simulink model "untitled"  (R2020a)
settings: Solver=VariableStepAuto  StartTime=0.0  StopTime=10.0  RelTol=1e-3
libraries: simulink_extras x1
settings Model: Creator=jiho  LastModifiedBy=jiho

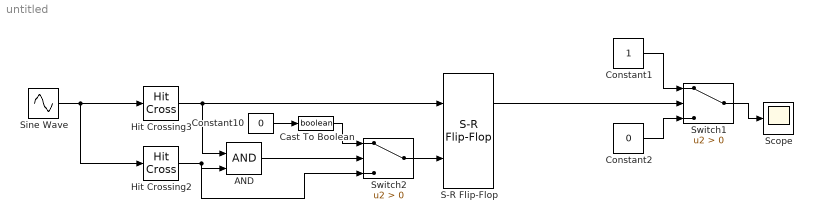
== system untitled ==
  AND : Logic  IconShape=distinctive  AllPortsSameDT=off  OutDataTypeStr=boolean
  Cast To Boolean : DataTypeConversion  OutDataTypeStr=boolean
  Constant1 : Constant
  Constant10 : Constant  Value=0
  Constant2 : Constant  Value=0
  Hit Crossing2 : HitCross  HitCrossingOffset=-0.5  HitCrossingDirection=rising
  Hit Crossing3 : HitCross  HitCrossingOffset=0.5  HitCrossingDirection=falling
  S-R Flip-Flop : simulink_extras/Flip Flops/S-R Flip-Flop  initial_condition=0
  Scope : Scope
  Sine Wave : Sin  SampleTime=0
  Switch1 : Switch  Criteria=u2 > Threshold
  Switch2 : Switch  Criteria=u2 > Threshold
  wires:
  Hit Crossing3/1 -> S-R Flip-Flop/1, AND/1
  Cast To Boolean/1 -> Switch2/1
  Hit Crossing2/1 -> Switch2/3, AND/2
  Constant1/1 -> Switch1/1
  Constant2/1 -> Switch1/3
  Switch2/1 -> S-R Flip-Flop/2
  S-R Flip-Flop/1 -> Switch1/2
  AND/1 -> Switch2/2
  Constant10/1 -> Cast To Boolean/1
  Sine Wave/1 -> Hit Crossing2/1, Hit Crossing3/1
  Switch1/1 -> Scope/1
